simulink model "asbhl20"  (R2016b)
settings: Solver=ode3  StartTime=0.0  StopTime=61  FixedStep=1/120  RelTol=1e-3  AbsTol=1e-6
PreLoadFcn:
  | load asbhl20data.mat
InitFcn:
  | timeSince1970.Value = etime(datevec(now),[1970, 1, 1, 0, 0, 0]);
values from neighbouring files (symbols this model uses):
  maxPackets = 100    [asbhl20data.mat]
  Tc = 0.0166666666667    [asbhl20GlobalChildrenData.mat]
  x_cg = 4.78635044684    [asbhl20data.mat]
undefined symbols (not defined in the file or in its folder): m, message, Receive, s, Send, sigbuilder_block
libraries: aerolibfltsims x5, simulink x4, asbhl20GPS x2, aerolibnav x2, asbhl20env x1, asbhl20airdata x1, asbhl20ralt x1, asbhl20commsys x1, asbhl20FADEC x1, asbhl20sensors x1, asbhl20LGC x1, asbhl20vehicle x1
(part 2 of 3)

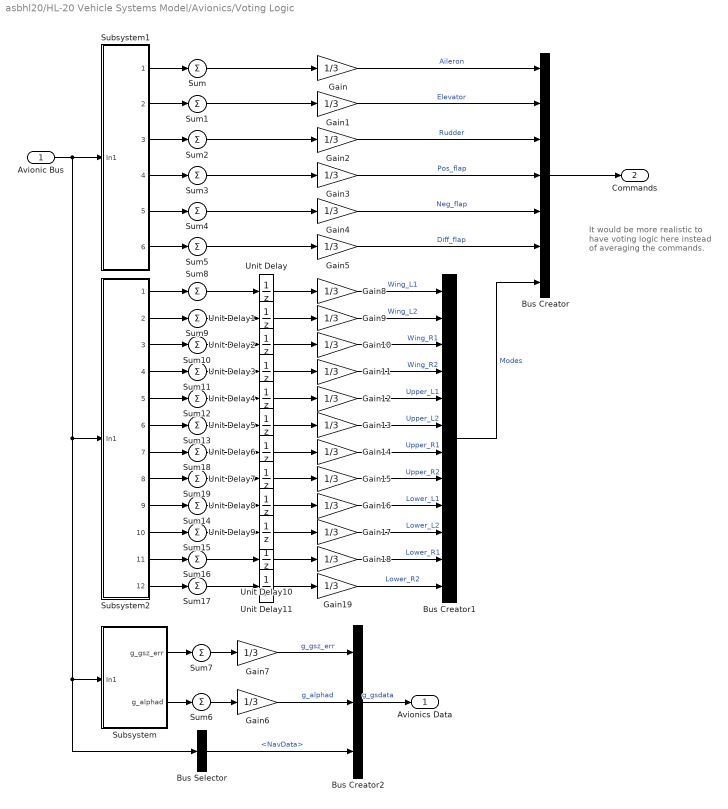
== system asbhl20/HL-20 Vehicle Systems Model/Avionics/Voting Logic ==
  note: It would be more realistic
      | to have voting logic here
      | instead of averaging the
      | commands.
  Avionic Bus : Inport
  Bus Creator : BusCreator  Inputs=7
  Bus Creator1 : BusCreator  Inputs=12
  Bus Creator2 : BusCreator  Inputs=3
  Bus Selector : BusSelector  OutputSignals=Bus1.CPU_A.NavData
  Gain{,1..7} (8 alike) : Gain  Gain=1/3  SaturateOnIntegerOverflow=on  OutDataTypeStr=Inherit: Same as input  ParamDataTypeStr=Inherit: Same as input
  Gain{8..19} (12 alike) : Gain  Gain=1/3  ParamDataTypeStr=float('double')  SaturateOnIntegerOverflow=on  OutDataTypeStr=Inherit: Same as input
  Subsystem : Subsystem
  Subsystem1 : Subsystem
  Subsystem2 : Subsystem
  Sum{,1..19} (20 alike) : Sum  Inputs=+  SaturateOnIntegerOverflow=on
  Unit Delay{,1..11} (12 alike) : UnitDelay  InitialCondition=12  SampleTime=Tc
  Avionics Data : Outport
  Commands : Outport  Port=2
  wires:
  Bus Creator1/1 -> Bus Creator/7  "Modes"
  Gain19/1 -> Bus Creator1/12  "Lower_R2"
  Gain18/1 -> Bus Creator1/11  "Lower_R1"
  Gain17/1 -> Bus Creator1/10  "Lower_L2"
  Gain16/1 -> Bus Creator1/9  "Lower_L1"
  Gain15/1 -> Bus Creator1/8  "Upper_R2"
  Gain14/1 -> Bus Creator1/7  "Upper_R1"
  Gain13/1 -> Bus Creator1/6  "Upper_L2"
  Gain12/1 -> Bus Creator1/5  "Upper_L1"
  Gain11/1 -> Bus Creator1/4  "Wing_R2"
  Gain10/1 -> Bus Creator1/3  "Wing_R1"
  Gain9/1 -> Bus Creator1/2  "Wing_L2"
  Gain8/1 -> Bus Creator1/1  "Wing_L1"
  Subsystem2/12(Lower_R2) -> Sum17/1
  Subsystem2/11(Lower_R1) -> Sum16/1
  Subsystem2/10(Lower_L2) -> Sum15/1
  Subsystem2/9(Lower_L1) -> Sum14/1
  Subsystem2/8(Upper_R2) -> Sum19/1
  Subsystem2/7(Upper_R1) -> Sum18/1
  Sum17/1 -> Unit Delay11/1
  Sum16/1 -> Unit Delay10/1
  Sum15/1 -> Unit Delay9/1
  Sum14/1 -> Unit Delay8/1
  Sum19/1 -> Unit Delay7/1
  Sum18/1 -> Unit Delay6/1
  Subsystem2/6(Upper_L2) -> Sum13/1
  Subsystem2/5(Upper_L1) -> Sum12/1
  Subsystem2/4(Wing_R2) -> Sum11/1
  Subsystem2/3(Wing_R1) -> Sum10/1
  Subsystem2/2(Wing_L2) -> Sum9/1
  Subsystem2/1(Wing_L1) -> Sum8/1
  Sum13/1 -> Unit Delay5/1
  Sum12/1 -> Unit Delay4/1
  Sum11/1 -> Unit Delay3/1
  Sum10/1 -> Unit Delay2/1
  Sum9/1 -> Unit Delay1/1
  Sum8/1 -> Unit Delay/1
  Subsystem/1("g_gsz_err ") -> Sum7/1
  Sum7/1 -> Gain7/1
  Subsystem/2("g_alphad ") -> Sum6/1
  Sum6/1 -> Gain6/1
  Gain6/1 -> Bus Creator2/2  "g_alphad"
  Gain7/1 -> Bus Creator2/1  "g_gsz_err"
  Bus Creator2/1 -> Avionics Data/1  "g_gsdata"
  Subsystem1/4(Pos Flap) -> Sum3/1
  Subsystem1/5(Neg Flap) -> Sum4/1
  Subsystem1/6(Diff Flap) -> Sum5/1
  Bus Creator/1 -> Commands/1
  Gain5/1 -> Bus Creator/6  "Diff_flap"
  Gain4/1 -> Bus Creator/5  "Neg_flap"
  Gain3/1 -> Bus Creator/4  "Pos_flap"
  Sum5/1 -> Gain5/1
  Sum4/1 -> Gain4/1
  Sum3/1 -> Gain3/1
  Gain2/1 -> Bus Creator/3  "Rudder"
  Subsystem1/3(Rudder) -> Sum2/1
  Sum2/1 -> Gain2/1
  Gain1/1 -> Bus Creator/2  "Elevator"
  Subsystem1/2(Elevator) -> Sum1/1
  Sum1/1 -> Gain1/1
  Subsystem1/1(Aileron) -> Sum/1
  Sum/1 -> Gain/1
  Avionic Bus/1 -> Subsystem2/1(In1), Subsystem/1(In1), Bus Selector/1, Subsystem1/1(In1)
  Gain/1 -> Bus Creator/1  "Aileron"
  Bus Selector/1 -> Bus Creator2/3  "<NavData>"
  Unit Delay/1 -> Gain8/1
  Unit Delay1/1 -> Gain9/1
  Unit Delay2/1 -> Gain10/1
  Unit Delay3/1 -> Gain11/1
  Unit Delay4/1 -> Gain12/1
  Unit Delay5/1 -> Gain13/1
  Unit Delay6/1 -> Gain14/1
  Unit Delay7/1 -> Gain15/1
  Unit Delay8/1 -> Gain16/1
  Unit Delay9/1 -> Gain17/1
  Unit Delay10/1 -> Gain18/1
  Unit Delay11/1 -> Gain19/1

== system asbhl20/Viewer and Feedback/FlightGear/Conditionally Receive net_ctrl Packet from FlightGear ==
  note: If FlightGear is not present or becomes unavailable, switch to pre-recorded data to avoid slowing the simulation due to repeated timeouts waiting for data that will not become available.
  Assertion : Assertion  AssertionFailFcn=warning(message('aeroblks:asbhl20:FGMaxPacketsLost'))  StopWhenAssertionFail=off
  Compare To Zero : simulink/Logic and Bit Operations/Compare To Zero  relop===  OutDataTypeStr=boolean
  Ground : Ground
  Memory : Memory  InheritSampleTime=on
  Pre-saved FlightGear data : Subsystem
      mask Display: port_label('output',1,sprintf('FG_data\n(Pre-saved)'))
  Self enabled subsystem receiving FlighGear data : Subsystem  TreatAsAtomicUnit=on
  Switch : Switch  Criteria=u2 ~= 0
  Switch1 : Switch  Criteria=u2 > Threshold
  Trigger a Warning Upon Loss of Connection : Logic  Operator=NAND  IconShape=distinctive  AllPortsSameDT=off  OutDataTypeStr=boolean
  Trigger signal : DiscretePulseGenerator  Period=4  SampleTime=1/120
  Env Data : Outport
  wires:
  Pre-saved FlightGear data/1(FG_data (Pre-saved)) -> Switch/1
  Switch/1 -> Env Data/1
  Compare To Zero/1 -> Trigger a Warning Upon Loss of Connection/1
  Memory/1 -> Compare To Zero/1, Switch1/2
  Ground/1 -> Switch1/1
  Switch1/1 -> Self enabled subsystem receiving FlighGear data/Trigger
  Trigger signal/1 -> Switch1/3
  Self enabled subsystem receiving FlighGear data/2(FGData) -> Switch/3
  Self enabled subsystem receiving FlighGear data/1(LostConn) -> Trigger a Warning Upon Loss of Connection/2, Memory/1, Switch/2
  Trigger a Warning Upon Loss of Connection/1 -> Assertion/1

== system asbhl20/Viewer and Feedback/FlightGear/phidot thetadot psidot ==
  pqr : Inport
  phi theta psi : Inport  Port=2
  Concatenate1 : Concatenate  NumInputs=3
  Concatenate2 : Concatenate  NumInputs=3
  SinCos : aerolibobsolete/SinCos
  phidot : Fcn  Expr=u[1]+(u[2]*u[4]+u[3]*u[7])*(u[5]/u[8])
  psidot : Fcn  Expr=(u[2]*u[4]+u[3]*u[7])/u[8]
  thetadot : Fcn  Expr=u[2]*u[7]-u[3]*u[4]
  ptp_earth : Outport
  ptp_dot : Outport  Port=2
  wires:
  SinCos/2 -> Concatenate1/3
  SinCos/1 -> Concatenate1/2
  Concatenate2/1 -> ptp_dot/1
  phidot/1 -> Concatenate2/1
  thetadot/1 -> Concatenate2/2
  psidot/1 -> Concatenate2/3
  phi theta psi/1 -> ptp_earth/1, SinCos/1
  pqr/1 -> Concatenate1/1
  Concatenate1/1 -> thetadot/1, phidot/1, psidot/1

== system asbhl20/Viewer and Feedback/Signal Builder/Signal Builder ==
  Demux : Demux  Tag=STV Demux  Outputs=8
  FromWs : FromWorkspace  Tag=STV FromWs  VariableName=tuvar  SampleTime=0
      SigBuilderData=|
      | common.afterFinalStr = 'Extrapolate'
      | common.sampleTime = 0
      | dataSet.timeRange = [0 10]
      | dataSet.name = 'Ramp Hold'
      | sbobj.Groups.Name = 'Ramp Hold'
      | sbobj.Groups.Signals(1).Name = 'wind_speed_kt'
      | sbobj.Groups.Signals(1).XData = [0 10]
      | sbobj.Groups.Signals(1).YData = [0 0]
      | sbobj.Groups.Signals(2).Name = 'wind_dir_deg'
      | sbobj.Groups.Signals(2).XData = [0 10]
      | sbobj.Groups.Signals(2).YData = [0 0]
      | sbobj.Groups.Signals(3).Name = 'turbulence_norm'
      | sbobj.Groups.Signals(3).XData = [0 10]
      | sbobj.Groups.Signals(3).YData = [0 0]
      | sbobj.Groups.Signals(4).Name = 'temp_c'
      | sbobj.Groups.Signals(4).XData = [0 10]
      | sbobj.Groups.Signals(4).YData = [-10 -10]
      | sbobj.Groups.Signals(5).Name = 'press_inhg'
      | sbobj.Groups.Signals(5).XData = [0 10]
      | sbobj.Groups.Signals(5).YData = [29.92 29.92]
      | sbobj.Groups.Signals(6).Name = 'hground'
      | sbobj.Groups.Signals(6).XData = [0 10]
      | sbobj.Groups.Signals(6).YData = [1 1]
      | sbobj.Groups.Signals(7).Name = 'magvar'
      | sbobj.Groups.Signals(7).XData = [0 10]
      | sbobj.Groups.Signals(7).YData = [0 0]
      | sbobj.Groups.Signals(8).Name = 'icing'
      | sbobj.Groups.Signals(8).XData = [0 10]
      | sbobj.Groups.Signals(8).YData = [0 0]
  wind_speed_kt : Outport  Tag=STV Outport
  wind_dir_deg : Outport  Tag=STV Outport  Port=2
  turbulence_norm : Outport  Tag=STV Outport  Port=3
  temp_c : Outport  Tag=STV Outport  Port=4
  press_inhg : Outport  Tag=STV Outport  Port=5
  hground : Outport  Tag=STV Outport  Port=6
  magvar : Outport  Tag=STV Outport  Port=7
  icing : Outport  Tag=STV Outport  Port=8
  wires:
  Demux/8 -> icing/1
  Demux/7 -> magvar/1
  Demux/6 -> hground/1
  Demux/5 -> press_inhg/1
  Demux/4 -> temp_c/1
  Demux/3 -> turbulence_norm/1
  Demux/2 -> wind_dir_deg/1
  Demux/1 -> wind_speed_kt/1
  FromWs/1 -> Demux/1

== system asbhl20/HL-20 Vehicle Systems Model/Avionics/Actuator System Failures /Left Lower Inner ==

== system asbhl20/HL-20 Vehicle Systems Model/Avionics/Actuator System Failures /Left Lower Outer ==

== system asbhl20/HL-20 Vehicle Systems Model/Avionics/Actuator System Failures /Left Upper Inner ==

== system asbhl20/HL-20 Vehicle Systems Model/Avionics/Actuator System Failures /Left Upper Outer ==

== system asbhl20/HL-20 Vehicle Systems Model/Avionics/Actuator System Failures /Right Lower Inner ==

== system asbhl20/HL-20 Vehicle Systems Model/Avionics/Actuator System Failures /Right Lower Outer ==

== system asbhl20/HL-20 Vehicle Systems Model/Avionics/Actuator System Failures /Right Upper Inner ==

== system asbhl20/HL-20 Vehicle Systems Model/Avionics/Actuator System Failures /Right Upper Outer ==

== system asbhl20/HL-20 Vehicle Systems Model/Avionics/Actuator System Failures /Wing H1 ==

== system asbhl20/HL-20 Vehicle Systems Model/Avionics/Actuator System Failures /Wing H2 ==

== system asbhl20/HL-20 Vehicle Systems Model/Avionics/Actuator System Failures /Wing H3 ==

== system asbhl20/HL-20 Vehicle Systems Model/Avionics/Actuator System Failures /Wing H4 ==

== system asbhl20/HL-20 Vehicle Systems Model/Avionics/Actuator System Failures /Wing H5 ==

== system asbhl20/HL-20 Vehicle Systems Model/Avionics/Actuator System Failures /Wing H6 ==

== system asbhl20/HL-20 Vehicle Systems Model/Avionics/Actuator System Failures /Wing H7 ==

== system asbhl20/HL-20 Vehicle Systems Model/Avionics/Actuator System Failures /Wing H8 ==

== system asbhl20/HL-20 Vehicle Systems Model/Avionics/Actuator System Failures /Wing H9 ==

== system asbhl20/HL-20 Vehicle Systems Model/Avionics/Actuator System Failures /Wing Left Inner ==

== system asbhl20/HL-20 Vehicle Systems Model/Avionics/Actuator System Failures /Wing Left Outer ==

== system asbhl20/HL-20 Vehicle Systems Model/Avionics/Actuator System Failures /Wing Right Inner ==

== system asbhl20/HL-20 Vehicle Systems Model/Avionics/Actuator System Failures /Wing Right Outer ==

== system asbhl20/HL-20 Vehicle Systems Model/Avionics/Left Avionics Bay/CPU B ==
  note: TODO: add redundant navigation application
  AirData : Inport
  Bus 2 : Inport  Port=2
  Bus 3 : Inport  Port=3
  Failures : Inport  Port=4
  Bus Creator1 : BusCreator  Inputs=4
  Bus Selector : BusSelector  OutputSignals=IMU2
  Bus Selector1 : BusSelector  OutputSignals=GPS2,h_sens
  Event Logging : Subsystem
  FDIR_Application : ModelReference  ModelNameDialog=asbhl20_FDIRApp  SimulationMode=Normal  ModelReferenceVersion=1.160
  FlightControlSystem_Application : ModelReference  ModelNameDialog=asbhl20_FCSApp  SimulationMode=Normal  ModelReferenceVersion=1.52
  GuidanceSystem_Application : ModelReference  ModelNameDialog=asbhl20_GuidanceApp  SimulationMode=Normal  ModelReferenceVersion=1.121
  IMU & GPS Post Process : Subsystem
  CPU_B_out : Outport
  wires:
  IMU & GPS Post Process/2(Guidance i/p) -> GuidanceSystem_Application/1
  IMU & GPS Post Process/1(Control i/p) -> FlightControlSystem_Application/2
  AirData/1 -> FDIR_Application/2, FlightControlSystem_Application/1, IMU & GPS Post Process/1(AirData)
  GuidanceSystem_Application/1 -> Bus Creator1/3, FlightControlSystem_Application/3  "Guidance"
  FlightControlSystem_Application/1 -> Bus Creator1/2  "Demands"
  Bus Creator1/1 -> CPU_B_out/1  "CPU_B"
  Bus Selector/1 -> IMU & GPS Post Process/2(IMU o/p)  "<IMU2>"
  Bus 3/1 -> Bus Selector/1
  Bus 2/1 -> Bus Selector1/1
  Bus Selector1/1 -> IMU & GPS Post Process/3(GPS o/p)  "<GPS2>"
  FDIR_Application/2 -> Bus Creator1/1  "Modes"
  FDIR_Application/1 -> Event Logging/1(Event_log)
  Failures/1 -> FDIR_Application/1
  Bus Selector1/2 -> IMU & GPS Post Process/4(NavData)  "<h_sens>"
  GuidanceSystem_Application/2 -> FlightControlSystem_Application/4
  GuidanceSystem_Application/3 -> Bus Creator1/4  "gsData"

== system asbhl20/HL-20 Vehicle Systems Model/Avionics/Left Avionics Bay/CPU C ==
  note: TODO: add redundant navigation application
  Airdata System o/p : Inport
  Bus 3 : Inport  Port=2
  Bus 1 : Inport  Port=3
  Failures : Inport  Port=4
  Average values : Subsystem
  Bus Creator1 : BusCreator  Inputs=4
  Bus Selector : BusSelector  OutputSignals=IMU2  OutputAsBus=on
  Bus Selector1 : BusSelector  OutputSignals=IMU1,GPS1,CPU_A.NavData
  Event Logging : Subsystem
  FDIR_Application : ModelReference  ModelNameDialog=asbhl20_FDIRApp  SimulationMode=Normal  ModelReferenceVersion=1.160
  FlightControlSystem_Application : ModelReference  ModelNameDialog=asbhl20_FCSApp  SimulationMode=Normal  ModelReferenceVersion=1.52
  GuidanceSystem_Application : ModelReference  ModelNameDialog=asbhl20_GuidanceApp  SimulationMode=Normal  ModelReferenceVersion=1.121
  IMU & GPS Post Process : Subsystem
  CPU_C_out : Outport
  wires:
  IMU & GPS Post Process/1(Control data) -> FlightControlSystem_Application/2
  Airdata System o/p/1 -> FDIR_Application/2, FlightControlSystem_Application/1, IMU & GPS Post Process/1(AirData)
  GuidanceSystem_Application/1 -> Bus Creator1/3, FlightControlSystem_Application/3  "Guidance"
  FlightControlSystem_Application/1 -> Bus Creator1/2  "Demands"
  Bus Creator1/1 -> CPU_C_out/1  "CPU_C"
  IMU & GPS Post Process/2(Guidance data) -> GuidanceSystem_Application/1
  Bus Selector/1 -> Average values/1(IMU2)
  Bus 3/1 -> Bus Selector/1
  Bus 1/1 -> Bus Selector1/1
  Bus Selector1/2 -> IMU & GPS Post Process/3(GPS o/p)  "<GPS1>"
  Bus Selector1/1 -> Average values/2(IMU1)  "<IMU1>"
  Average values/1(IMUave) -> IMU & GPS Post Process/2(IMU o/p)
  FDIR_Application/2 -> Bus Creator1/1  "Modes"
  FDIR_Application/1 -> Event Logging/1(Event_log)
  Failures/1 -> FDIR_Application/1
  Bus Selector1/3 -> IMU & GPS Post Process/4(NavData)  "<NavData>"
  GuidanceSystem_Application/2 -> FlightControlSystem_Application/4
  GuidanceSystem_Application/3 -> Bus Creator1/4  "gsData"

== system asbhl20/HL-20 Vehicle Systems Model/Avionics/Left Avionics Bay/bus comm delay ==
  note: TODO: resolve Demands as a bus
  curr : Inport
  Bus Creator2 : BusCreator  Inputs=3
  Bus Selector3 : BusSelector  OutputSignals=Demands,Guidance,NavData
  Unit Delay1 : UnitDelay  SampleTime=Tc
  Unit Delay7 : UnitDelay  SampleTime=Tc
  Unit Delay8 : UnitDelay  SampleTime=Tc
  prev : Outport
  wires:
  Unit Delay7/1 -> Bus Creator2/2  "Guidance_out"
  Bus Selector3/2 -> Unit Delay7/1  "<Guidance>"
  curr/1 -> Bus Selector3/1
  Bus Selector3/1 -> Unit Delay8/1  "<Demands>"
  Unit Delay8/1 -> Bus Creator2/1  "Demands"
  Bus Creator2/1 -> prev/1
  Bus Selector3/3 -> Unit Delay1/1  "<NavData>"
  Unit Delay1/1 -> Bus Creator2/3  "NavData"

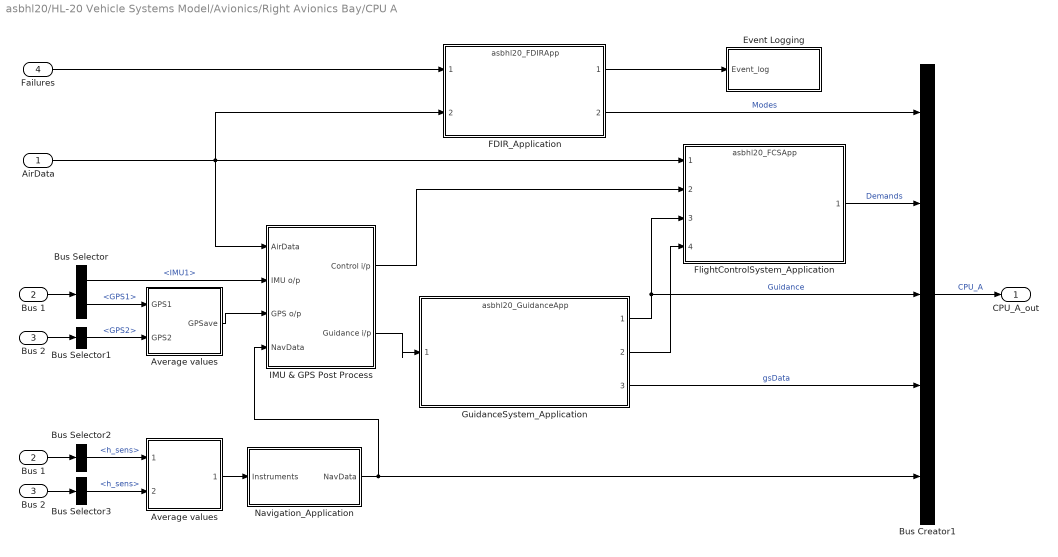
== system asbhl20/HL-20 Vehicle Systems Model/Avionics/Right Avionics Bay/CPU A ==
  AirData : Inport
  Bus 1 : Inport  Port=2
  Bus 2 : Inport  Port=3
  Failures : Inport  Port=4
  Average values : Subsystem
  "Average values " : Subsystem
  Bus Creator1 : BusCreator  Inputs=5
  Bus Selector : BusSelector  OutputSignals=IMU1,GPS1
  Bus Selector1 : BusSelector  OutputSignals=GPS2
  Bus Selector2 : BusSelector  OutputSignals=h_sens
  Bus Selector3 : BusSelector  OutputSignals=h_sens
  "Bus 1 " : InportShadow  Port=2
  "Bus 2 " : InportShadow  Port=3
  Event Logging : Subsystem
  FDIR_Application : ModelReference  ModelNameDialog=asbhl20_FDIRApp  SimulationMode=Normal  ModelReferenceVersion=1.160
  FlightControlSystem_Application : ModelReference  ModelNameDialog=asbhl20_FCSApp  SimulationMode=Normal  ModelReferenceVersion=1.52
  GuidanceSystem_Application : ModelReference  ModelNameDialog=asbhl20_GuidanceApp  SimulationMode=Normal  ModelReferenceVersion=1.121
  IMU & GPS Post Process : Subsystem
  Navigation_Application : Subsystem  TreatAsAtomicUnit=on
  CPU_A_out : Outport
  wires:
  FlightControlSystem_Application/1 -> Bus Creator1/2  "Demands"
  GuidanceSystem_Application/1 -> FlightControlSystem_Application/3, Bus Creator1/3  "Guidance"
  AirData/1 -> IMU & GPS Post Process/1(AirData), FDIR_Application/2, FlightControlSystem_Application/1
  IMU & GPS Post Process/1(Control i/p) -> FlightControlSystem_Application/2
  IMU & GPS Post Process/2(Guidance i/p) -> GuidanceSystem_Application/1
  Bus Creator1/1 -> CPU_A_out/1  "CPU_A"
  Bus Selector/1 -> IMU & GPS Post Process/2(IMU o/p)  "<IMU1>"
  Bus 1/1 -> Bus Selector/1
  Bus 2/1 -> Bus Selector1/1
  Bus Selector1/1 -> Average values/2(GPS2)  "<GPS2>"
  Average values/1(GPSave) -> IMU & GPS Post Process/3(GPS o/p)
  Bus Selector/2 -> Average values/1(GPS1)  "<GPS1>"
  "Bus 1 "/1 -> Bus Selector2/1
  "Bus 2 "/1 -> Bus Selector3/1
  Bus Selector2/1 -> "Average values "/1(h_sens1)  "<h_sens>"
  Bus Selector3/1 -> "Average values "/2(h_sens2)  "<h_sens>"
  "Average values "/1(h_sens_avg) -> Navigation_Application/1(Instruments)
  Navigation_Application/1(NavData) -> Bus Creator1/5, IMU & GPS Post Process/4(NavData)
  FDIR_Application/2 -> Bus Creator1/1  "Modes"
  FDIR_Application/1 -> Event Logging/1(Event_log)
  Failures/1 -> FDIR_Application/1
  GuidanceSystem_Application/2 -> FlightControlSystem_Application/4
  GuidanceSystem_Application/3 -> Bus Creator1/4  "gsData"

== system asbhl20/HL-20 Vehicle Systems Model/Avionics/Right Avionics Bay/bus comm delay ==
  note: TODO: resolve Demands as a bus
  curr : Inport
  Bus Creator2 : BusCreator  Inputs=2
  Bus Selector3 : BusSelector  OutputSignals=Demands,Guidance
  Unit Delay7 : UnitDelay  SampleTime=Tc
  Unit Delay8 : UnitDelay  SampleTime=Tc
  prev : Outport
  wires:
  Unit Delay7/1 -> Bus Creator2/2  "Guidance_out"
  Bus Selector3/2 -> Unit Delay7/1  "<Guidance>"
  curr/1 -> Bus Selector3/1
  Bus Selector3/1 -> Unit Delay8/1  "<Demands>"
  Unit Delay8/1 -> Bus Creator2/1  "Demands"
  Bus Creator2/1 -> prev/1

== system asbhl20/HL-20 Vehicle Systems Model/Avionics/Voting Logic/Subsystem ==
  In1 : Inport
  Bus Selector1 : BusSelector  OutputSignals=Bus1.CPU_A.gsData,Bus2.CPU_B.gsData,Bus3.CPU_C.gsData
  Bus to Vector : BusToVector
  Bus to Vector1 : BusToVector
  Bus to Vector2 : BusToVector
  Mux9 : Mux  Inputs=[2 2 2]
  g_alphad : Selector  InputPortWidth=6  IndexOptions=Index vector (dialog)  Indices=[2 4 6]  OutputSizes=1
  g_gsz_err : Selector  InputPortWidth=6  IndexOptions=Index vector (dialog)  Indices=[1 3 5]  OutputSizes=1
  "g_gsz_err " : Outport
  "g_alphad " : Outport  Port=2
  wires:
  g_alphad/1 -> "g_alphad "/1
  In1/1 -> Bus Selector1/1
  g_gsz_err/1 -> "g_gsz_err "/1
  Bus Selector1/1 -> Bus to Vector/1  "<gsData>"
  Bus Selector1/3 -> Bus to Vector2/1  "<gsData>"
  Bus Selector1/2 -> Bus to Vector1/1  "<gsData>"
  Mux9/1 -> g_alphad/1, g_gsz_err/1
  Bus to Vector/1 -> Mux9/1
  Bus to Vector1/1 -> Mux9/2
  Bus to Vector2/1 -> Mux9/3

== system asbhl20/HL-20 Vehicle Systems Model/Avionics/Voting Logic/Subsystem1 ==
  In1 : Inport
  Bus Selector1 : BusSelector  OutputSignals=Bus1.CPU_A.Demands.Aileron_demand,Bus2.CPU_B.Demands.Aileron_demand,Bus3.CPU_C.Demands.Aileron_demand,Bus1.CPU_A.Demands.Elevator_demand,Bus2.CPU_B.Demands.Elevator_demand,Bus3.CPU_C.Demands.Elevator_demand,Bus1.CPU_A.Demands.Rudder_demand,Bus2.CPU_B.Demands.Rudder_demand,Bus3.CPU_C.Demands.Rudder_demand,Bus1.CPU_A.Demands.Positive_flap_demand,Bus2.CPU_B.Demands.Positive_flap_demand,Bus3.CPU_C.Demands.Positive_flap_demand,Bus1.CPU_A.Demands.Negative_flap_demand,Bus2.CPU_B.Demands.Negative_flap_demand,Bus3.CPU_C.Demands.Negative_flap_demand,Bus1.CPU_A.Demands.Differential_flap_demand,Bus2.CPU_B.Demands.Differential_flap_demand,Bus3.CPU_C.Demands.Differential_flap_demand
  Mux{,1..5} (6 alike) : Mux  Inputs=3
  Aileron : Outport
  Elevator : Outport  Port=2
  Rudder : Outport  Port=3
  Pos Flap : Outport  Port=4
  Neg Flap : Outport  Port=5
  Diff Flap : Outport  Port=6
  wires:
  Mux5/1 -> Diff Flap/1
  Mux4/1 -> Neg Flap/1
  Mux3/1 -> Pos Flap/1
  In1/1 -> Bus Selector1/1
  Mux2/1 -> Rudder/1
  Mux1/1 -> Elevator/1
  Mux/1 -> Aileron/1
  Bus Selector1/1 -> Mux/1  "<Aileron_demand>"
  Bus Selector1/2 -> Mux/2  "<Aileron_demand>"
  Bus Selector1/3 -> Mux/3  "<Aileron_demand>"
  Bus Selector1/4 -> Mux1/1  "<Elevator_demand>"
  Bus Selector1/5 -> Mux1/2  "<Elevator_demand>"
  Bus Selector1/6 -> Mux1/3  "<Elevator_demand>"
  Bus Selector1/7 -> Mux2/1  "<Rudder_demand>"
  Bus Selector1/8 -> Mux2/2  "<Rudder_demand>"
  Bus Selector1/9 -> Mux2/3  "<Rudder_demand>"
  Bus Selector1/10 -> Mux3/1  "<Positive_flap_demand>"
  Bus Selector1/11 -> Mux3/2  "<Positive_flap_demand>"
  Bus Selector1/12 -> Mux3/3  "<Positive_flap_demand>"
  Bus Selector1/13 -> Mux4/1  "<Negative_flap_demand>"
  Bus Selector1/14 -> Mux4/2  "<Negative_flap_demand>"
  Bus Selector1/15 -> Mux4/3  "<Negative_flap_demand>"
  Bus Selector1/16 -> Mux5/1  "<Differential_flap_demand>"
  Bus Selector1/17 -> Mux5/2  "<Differential_flap_demand>"
  Bus Selector1/18 -> Mux5/3  "<Differential_flap_demand>"

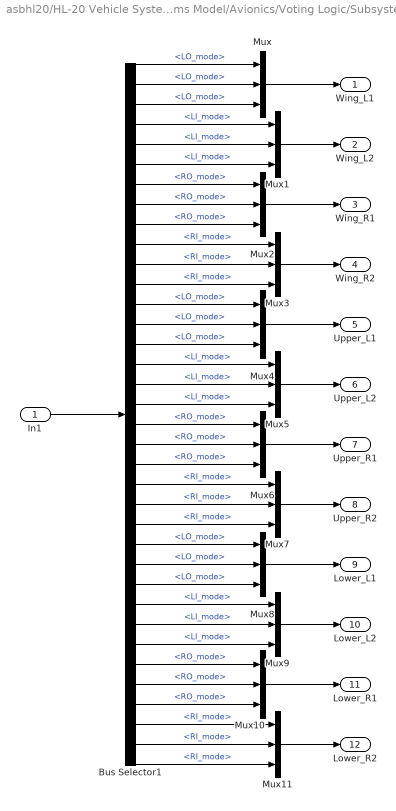
== system asbhl20/HL-20 Vehicle Systems Model/Avionics/Voting Logic/Subsystem2 ==
  In1 : Inport
  Bus Selector1 : BusSelector  OutputSignals=Bus1.CPU_A.Modes.Wing.LO_mode,Bus2.CPU_B.Modes.Wing.LO_mode,Bus3.CPU_C.Modes.Wing.LO_mode,Bus1.CPU_A.Modes.Wing.LI_mode,Bus2.CPU_B.Modes.Wing.LI_mode,Bus3.CPU_C.Modes.Wing.LI_mode,Bus1.CPU_A.Modes.Wing.RO_mode,Bus2.CPU_B.Modes.Wing.RO_mode,Bus3.CPU_C.Modes.Wing.RO_mode,Bus1.CPU_A.Modes.Wing.RI_mode,Bus2.CPU_B.Modes.Wing.RI_mode,Bus3.CPU_C.Modes.Wing.RI_mode,Bus1.CPU_A.Modes.Upper.LO_mode,Bus2.CPU_B.Modes.Upper.LO_mode,Bus3.CPU_C.Modes.Upper.LO_mode,Bus1.CPU_A.Modes.Upper.LI_mode,Bus2.CPU_B.Modes.Upper.LI_mode,Bus3.CPU_C.Modes.Upper.LI_mode,Bus1.CPU_A.Modes.Upper.RO_mode,Bus2.CPU_B.Modes.Upper.RO_mode,Bus3.CPU_C.Modes.Upper.RO_mode,Bus1.CPU_A.Modes.Upper.RI_mode,Bus2.CPU_B.Modes.Upper.RI_mode,Bus3.CPU_C.Modes.Upper.RI_mode,Bus1.CPU_A.Modes.Lower.LO_mode,Bus2.CPU_B.Modes.Lower.LO_mode,Bus3.CPU_C.Modes.Lower.LO_mode,Bus1.CPU_A.Modes.Lower.LI_mode,Bus2.CPU_B.Modes.Lower.LI_mode,Bus3.CPU_C.Modes.Lower.LI_mode,Bus1.CPU_A.Modes.Lower.RO_mode,Bus2.CPU_B.Modes.Lower.RO_mode,Bus3.CPU_C.Modes.Lower.RO_mode,Bus1.CPU_A.Modes.Lower.RI_mode,Bus2.CPU_B.Modes.Lower.RI_mode,Bus3.CPU_C.Modes.Lower.RI_mode
  Mux{,1..11} (12 alike) : Mux  Inputs=3
  Wing_L1 : Outport
  Wing_L2 : Outport  Port=2
  Wing_R1 : Outport  Port=3
  Wing_R2 : Outport  Port=4
  Upper_L1 : Outport  Port=5
  Upper_L2 : Outport  Port=6
  Upper_R1 : Outport  Port=7
  Upper_R2 : Outport  Port=8
  Lower_L1 : Outport  Port=9
  Lower_L2 : Outport  Port=10
  Lower_R1 : Outport  Port=11
  Lower_R2 : Outport  Port=12
  wires:
  Mux11/1 -> Lower_R2/1
  Mux10/1 -> Lower_R1/1
  Mux9/1 -> Lower_L2/1
  Mux8/1 -> Lower_L1/1
  Mux7/1 -> Upper_R2/1
  Mux6/1 -> Upper_R1/1
  Bus Selector1/36 -> Mux11/3  "<RI_mode>"
  Bus Selector1/35 -> Mux11/2  "<RI_mode>"
  Bus Selector1/34 -> Mux11/1  "<RI_mode>"
  Bus Selector1/33 -> Mux10/3  "<RO_mode>"
  Bus Selector1/32 -> Mux10/2  "<RO_mode>"
  Bus Selector1/31 -> Mux10/1  "<RO_mode>"
  Bus Selector1/30 -> Mux9/3  "<LI_mode>"
  Bus Selector1/29 -> Mux9/2  "<LI_mode>"
  Bus Selector1/28 -> Mux9/1  "<LI_mode>"
  Bus Selector1/27 -> Mux8/3  "<LO_mode>"
  Bus Selector1/26 -> Mux8/2  "<LO_mode>"
  Bus Selector1/25 -> Mux8/1  "<LO_mode>"
  Bus Selector1/24 -> Mux7/3  "<RI_mode>"
  Bus Selector1/23 -> Mux7/2  "<RI_mode>"
  Bus Selector1/22 -> Mux7/1  "<RI_mode>"
  Bus Selector1/21 -> Mux6/3  "<RO_mode>"
  Bus Selector1/20 -> Mux6/2  "<RO_mode>"
  Bus Selector1/19 -> Mux6/1  "<RO_mode>"
  Bus Selector1/18 -> Mux5/3  "<LI_mode>"
  Bus Selector1/17 -> Mux5/2  "<LI_mode>"
  Bus Selector1/16 -> Mux5/1  "<LI_mode>"
  Bus Selector1/15 -> Mux4/3  "<LO_mode>"
  Bus Selector1/14 -> Mux4/2  "<LO_mode>"
  Bus Selector1/13 -> Mux4/1  "<LO_mode>"
  Bus Selector1/12 -> Mux3/3  "<RI_mode>"
  Bus Selector1/11 -> Mux3/2  "<RI_mode>"
  Bus Selector1/10 -> Mux3/1  "<RI_mode>"
  Bus Selector1/9 -> Mux2/3  "<RO_mode>"
  Bus Selector1/8 -> Mux2/2  "<RO_mode>"
  Bus Selector1/7 -> Mux2/1  "<RO_mode>"
  Bus Selector1/6 -> Mux1/3  "<LI_mode>"
  Bus Selector1/5 -> Mux1/2  "<LI_mode>"
  Bus Selector1/4 -> Mux1/1  "<LI_mode>"
  Bus Selector1/3 -> Mux/3  "<LO_mode>"
  Bus Selector1/2 -> Mux/2  "<LO_mode>"
  Bus Selector1/1 -> Mux/1  "<LO_mode>"
  Mux/1 -> Wing_L1/1
  Mux1/1 -> Wing_L2/1
  Mux2/1 -> Wing_R1/1
  In1/1 -> Bus Selector1/1
  Mux3/1 -> Wing_R2/1
  Mux4/1 -> Upper_L1/1
  Mux5/1 -> Upper_L2/1

== system asbhl20/Viewer and Feedback/FlightGear/Conditionally Receive net_ctrl Packet from FlightGear/Pre-saved FlightGear data ==
  Bus Creator2 : BusCreator  Inputs=8  OutDataTypeStr=Bus: FlightGearBus
  Data Type Conversion : DataTypeConversion  OutDataTypeStr=uint32
  Demux2 : Demux  Outputs=8
  From File : FromFile  FileName=asbhl20FlightGear.mat  SampleTime=1/120
  FG_data (Pre-saved) : Outport
  wires:
  From File/1 -> Demux2/1
  Demux2/6 -> Bus Creator2/6  "hground"
  Data Type Conversion/1 -> Bus Creator2/8  "icing"
  Demux2/7 -> Bus Creator2/7  "magvar"
  Demux2/4 -> Bus Creator2/4  "temp_c"
  Demux2/3 -> Bus Creator2/3  "turbulence_norm"
  Demux2/2 -> Bus Creator2/2  "wind_dir_deg"
  Demux2/1 -> Bus Creator2/1  "wind_speed_kt"
  Demux2/8 -> Data Type Conversion/1
  Demux2/5 -> Bus Creator2/5  "press_inhg"
  Bus Creator2/1 -> FG_data (Pre-saved)/1

== system asbhl20/Viewer and Feedback/FlightGear/Conditionally Receive net_ctrl Packet from FlightGear/Self enabled subsystem receiving FlighGear data ==
  Trigger : TriggerPort  VariantControl=Variant
  Bias : Bias  Bias=1
  Bus Creator1 : BusCreator  Inputs=8  OutDataTypeStr=Bus: FlightGearBus
  Compare To Constant : simulink/Logic and Bit Operations/Compare To Constant  relop=>=  const=maxPackets  OutDataTypeStr=boolean
  Constant : Constant  Value=0
  Memory : Memory  InheritSampleTime=on
  Receive net_ctrl Packet from FlightGear : aerolibfltsims/Receive net_ctrl Packet from FlightGear  FlightGearVersion=v2016.1  ReceiveAddress=127.0.0.1  ReceivePort=5505  ReceiveWidth=744  varLen=off  SampleTime=-1  packetFlag=on
      settings: AttributesFormatString=Version Selected:\n%<FlightGearVersion>
  Switch : Switch  Criteria=u2 > Threshold
  Unpack net_ctrl Packet from FlightGear : aerolibfltsims/Unpack net_ctrl Packet from FlightGear  FlightGearVersion=v2016.1  ShowControlSurfacePositionOutputs=off  ShowEngineFuelOutputs=off  ShowLandingGearOutputs=off  ShowAvionicOutputs=off  ShowEnvironmentOutputs=on  SampleTime=-1
      settings: AttributesFormatString=Version Selected: %<FlightGearVersion>
  LostConn : Outport  InitialOutput=0
  FGData : Outport  Port=2
  wires:
  Receive net_ctrl Packet from FlightGear/2 -> Switch/2
  Switch/1 -> Memory/1, Compare To Constant/1
  Bias/1 -> Switch/3
  Constant/1 -> Switch/1
  Memory/1 -> Bias/1
  Compare To Constant/1 -> LostConn/1
  Unpack net_ctrl Packet from FlightGear/6 -> Bus Creator1/6  "hground"
  Unpack net_ctrl Packet from FlightGear/8 -> Bus Creator1/8  "icing"
  Unpack net_ctrl Packet from FlightGear/7 -> Bus Creator1/7  "magvar"
  Unpack net_ctrl Packet from FlightGear/5 -> Bus Creator1/5  "press_inhg"
  Unpack net_ctrl Packet from FlightGear/4 -> Bus Creator1/4  "temp_c"
  Unpack net_ctrl Packet from FlightGear/3 -> Bus Creator1/3  "turbulence_norm"
  Unpack net_ctrl Packet from FlightGear/2 -> Bus Creator1/2  "wind_dir_deg"
  Unpack net_ctrl Packet from FlightGear/1 -> Bus Creator1/1  "wind_speed_kt"
  Receive net_ctrl Packet from FlightGear/1 -> Unpack net_ctrl Packet from FlightGear/1
  Bus Creator1/1 -> FGData/1

== system asbhl20/HL-20 Vehicle Systems Model/Avionics/Left Avionics Bay/CPU B/Event Logging ==
  Event_log : Inport
  Bus Selector : BusSelector  OutputSignals=Left_log,Right_log,Wing_log,WingH_log,UpperH_log,LowerH_log
  Event Logging Left : Subsystem
  Event Logging Lower Hydraulic : Subsystem
  Event Logging Right : Subsystem
  Event Logging Upper Hydraulic : Subsystem
  Event Logging Wing : Subsystem
  Event Logging Wing Hydraulic : Subsystem
  wires:
  Event_log/1 -> Bus Selector/1
  Bus Selector/1 -> Event Logging Left/1(In1)  "<Left_log>"
  Bus Selector/2 -> Event Logging Right/1(In1)  "<Right_log>"
  Bus Selector/3 -> Event Logging Wing/1(In1)  "<Wing_log>"
  Bus Selector/4 -> Event Logging Wing Hydraulic/1(In1)  "<WingH_log>"
  Bus Selector/5 -> Event Logging Upper Hydraulic/1(In1)  "<UpperH_log>"
  Bus Selector/6 -> Event Logging Lower Hydraulic/1(In1)  "<LowerH_log>"

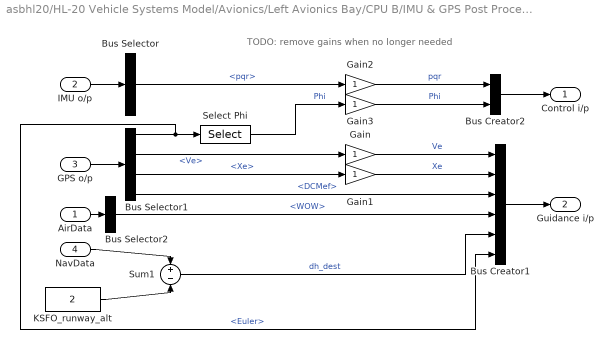
== system asbhl20/HL-20 Vehicle Systems Model/Avionics/Left Avionics Bay/CPU B/IMU & GPS Post Process ==
  note: TODO: remove gains when no longer needed
  AirData : Inport
  IMU o/p : Inport  Port=2
  GPS o/p : Inport  Port=3
  NavData : Inport  Port=4
  Bus Creator1 : BusCreator  Inputs=6  OutDataTypeStr=Bus: GuidanceBus
  Bus Creator2 : BusCreator  Inputs=2  OutDataTypeStr=Bus: FCSSensorBus
  Bus Selector : BusSelector  OutputSignals=pqr
  Bus Selector1 : BusSelector  OutputSignals=Euler,Ve,Xe,DCMef
  Bus Selector2 : BusSelector  OutputSignals=WOW
  Gain{,1..3} (4 alike) : Gain
  KSFO_runway_alt : Constant  Value=2  SampleTime=Tc
  Select Phi : Selector  InputPortWidth=3  IndexOptions=Index vector (dialog)  Indices=[1]  OutputSizes=1
  Sum1 : Sum  Inputs=+-
  Control i/p : Outport
  Guidance i/p : Outport  Port=2
  wires:
  GPS o/p/1 -> Bus Selector1/1
  IMU o/p/1 -> Bus Selector/1
  Bus Creator1/1 -> Guidance i/p/1
  Select Phi/1 -> Gain3/1  "Phi"
  Bus Creator2/1 -> Control i/p/1
  Bus Selector/1 -> Gain2/1  "<pqr>"
  Bus Selector1/3 -> Gain1/1  "<Xe>"
  Bus Selector1/1 -> Select Phi/1, Bus Creator1/6  "<Euler>"
  Bus Selector1/2 -> Gain/1  "<Ve>"
  AirData/1 -> Bus Selector2/1
  Bus Selector2/1 -> Bus Creator1/4  "<WOW>"
  Gain/1 -> Bus Creator1/1  "Ve"
  Gain1/1 -> Bus Creator1/2  "Xe"
  Gain2/1 -> Bus Creator2/1  "pqr"
  Gain3/1 -> Bus Creator2/2  "Phi"
  Bus Selector1/4 -> Bus Creator1/3  "<DCMef>"
  NavData/1 -> Sum1/1
  Sum1/1 -> Bus Creator1/5  "dh_dest"
  KSFO_runway_alt/1 -> Sum1/2

== system asbhl20/HL-20 Vehicle Systems Model/Avionics/Left Avionics Bay/CPU C/Average values ==
  IMU2 : Inport
  IMU1 : Inport  Port=2
  Bus Creator1 : BusCreator  Inputs=1
  Bus Selector : BusSelector  OutputSignals=pqr
  Bus Selector1 : BusSelector  OutputSignals=pqr
  Gain : Gain  Gain=0.5  SaturateOnIntegerOverflow=on  OutDataTypeStr=Inherit: Same as input  ParamDataTypeStr=Inherit: Same as input
  Sum : Sum  Inputs=+|+  SaturateOnIntegerOverflow=on
  IMUave : Outport
  wires:
  IMU1/1 -> Bus Selector/1
  Sum/1 -> Gain/1
  IMU2/1 -> Bus Selector1/1
  Bus Selector1/1 -> Sum/1  "<pqr>"
  Bus Selector/1 -> Sum/2  "<pqr>"
  Gain/1 -> Bus Creator1/1  "pqr"
  Bus Creator1/1 -> IMUave/1

== system asbhl20/HL-20 Vehicle Systems Model/Avionics/Left Avionics Bay/CPU C/Event Logging ==
  Event_log : Inport
  Bus Selector : BusSelector  OutputSignals=Left_log,Right_log,Wing_log,WingH_log,UpperH_log,LowerH_log
  Event Logging Left : Subsystem
  Event Logging Lower Hydraulic : Subsystem
  Event Logging Right : Subsystem
  Event Logging Upper Hydraulic : Subsystem
  Event Logging Wing : Subsystem
  Event Logging Wing Hydraulic : Subsystem
  wires:
  Event_log/1 -> Bus Selector/1
  Bus Selector/1 -> Event Logging Left/1(In1)  "<Left_log>"
  Bus Selector/2 -> Event Logging Right/1(In1)  "<Right_log>"
  Bus Selector/3 -> Event Logging Wing/1(In1)  "<Wing_log>"
  Bus Selector/4 -> Event Logging Wing Hydraulic/1(In1)  "<WingH_log>"
  Bus Selector/5 -> Event Logging Upper Hydraulic/1(In1)  "<UpperH_log>"
  Bus Selector/6 -> Event Logging Lower Hydraulic/1(In1)  "<LowerH_log>"

== system asbhl20/HL-20 Vehicle Systems Model/Avionics/Left Avionics Bay/CPU C/IMU & GPS Post Process ==
  note: TODO: resolve signals without gain-of-1
  AirData : Inport
  IMU o/p : Inport  Port=2
  GPS o/p : Inport  Port=3
  NavData : Inport  Port=4
  Bus Creator2 : BusCreator  Inputs=2  OutDataTypeStr=Bus: FCSSensorBus
  Bus Creator3 : BusCreator  Inputs=6  OutDataTypeStr=Bus: GuidanceBus
  Bus Selector : BusSelector  OutputSignals=pqr
  Bus Selector1 : BusSelector  OutputSignals=Euler,Ve,Xe,DCMef
  Bus Selector2 : BusSelector  OutputSignals=WOW
  Bus Selector3 : BusSelector  OutputSignals=dh_dest
  Gain{,1..3} (4 alike) : Gain
  Select Phi : Selector  InputPortWidth=3  IndexOptions=Index vector (dialog)  Indices=[1]  OutputSizes=1
  Control data : Outport
  Guidance data : Outport  Port=2
  wires:
  GPS o/p/1 -> Bus Selector1/1
  IMU o/p/1 -> Bus Selector/1
  Bus Creator3/1 -> Guidance data/1
  Select Phi/1 -> Gain3/1  "Phi"
  Bus Creator2/1 -> Control data/1
  Bus Selector/1 -> Gain2/1  "<pqr>"
  Bus Selector1/3 -> Gain1/1  "<Xe>"
  Bus Selector1/1 -> Bus Creator3/6, Select Phi/1  "<Euler>"
  Bus Selector1/2 -> Gain/1  "<Ve>"
  AirData/1 -> Bus Selector2/1
  Bus Selector2/1 -> Bus Creator3/4  "<WOW>"
  Gain/1 -> Bus Creator3/1  "Ve"
  Gain1/1 -> Bus Creator3/2  "Xe"
  Gain2/1 -> Bus Creator2/1  "pqr"
  Gain3/1 -> Bus Creator2/2  "Phi"
  Bus Selector1/4 -> Bus Creator3/3  "<DCMef>"
  NavData/1 -> Bus Selector3/1
  Bus Selector3/1 -> Bus Creator3/5  "<dh_dest>"

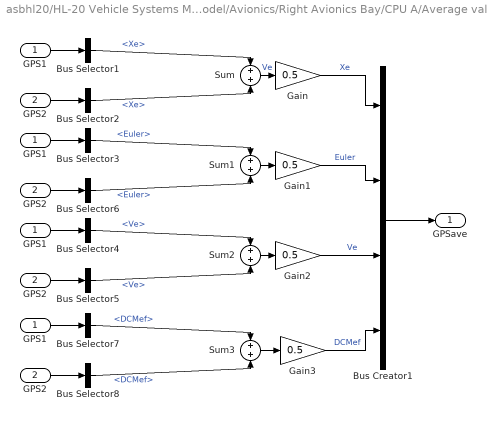
== system asbhl20/HL-20 Vehicle Systems Model/Avionics/Right Avionics Bay/CPU A/Average values ==
  GPS1 : Inport
  GPS2 : Inport  Port=2
  " GPS1" : InportShadow
  " GPS1 " : InportShadow
  " GPS2" : InportShadow  Port=2
  " GPS2 " : InportShadow  Port=2
  Bus Creator1 : BusCreator  Inputs=4
  Bus Selector1 : BusSelector  OutputSignals=Xe
  Bus Selector2 : BusSelector  OutputSignals=Xe
  Bus Selector3 : BusSelector  OutputSignals=Euler
  Bus Selector4 : BusSelector  OutputSignals=Ve
  Bus Selector5 : BusSelector  OutputSignals=Ve
  Bus Selector6 : BusSelector  OutputSignals=Euler
  Bus Selector7 : BusSelector  OutputSignals=DCMef
  Bus Selector8 : BusSelector  OutputSignals=DCMef
  "GPS1 " : InportShadow
  "GPS2 " : InportShadow  Port=2
  Gain{,1..3} (4 alike) : Gain  Gain=0.5  SaturateOnIntegerOverflow=on  OutDataTypeStr=Inherit: Same as input  ParamDataTypeStr=Inherit: Same as input
  Sum{,1..3} (4 alike) : Sum  Inputs=+|+  SaturateOnIntegerOverflow=on
  GPSave : Outport
  wires:
  GPS2/1 -> Bus Selector2/1
  Sum/1 -> Gain/1  "Ve"
  GPS1/1 -> Bus Selector1/1
  Bus Creator1/1 -> GPSave/1
  Sum1/1 -> Gain1/1
  Gain1/1 -> Bus Creator1/2  "Euler"
  Gain/1 -> Bus Creator1/1  "Xe"
  Bus Selector1/1 -> Sum/1  "<Xe>"
  Bus Selector2/1 -> Sum/2  "<Xe>"
  Sum2/1 -> Gain2/1
  Gain2/1 -> Bus Creator1/3  "Ve"
  "GPS1 "/1 -> Bus Selector3/1
  Bus Selector3/1 -> Sum1/1  "<Euler>"
  " GPS1"/1 -> Bus Selector4/1
  Bus Selector4/1 -> Sum2/1  "<Ve>"
  " GPS2"/1 -> Bus Selector5/1
  Bus Selector5/1 -> Sum2/2  "<Ve>"
  "GPS2 "/1 -> Bus Selector6/1
  Bus Selector6/1 -> Sum1/2  "<Euler>"
  " GPS1 "/1 -> Bus Selector7/1
  Bus Selector7/1 -> Sum3/1  "<DCMef>"
  " GPS2 "/1 -> Bus Selector8/1
  Bus Selector8/1 -> Sum3/2  "<DCMef>"
  Sum3/1 -> Gain3/1
  Gain3/1 -> Bus Creator1/4  "DCMef"

== system asbhl20/HL-20 Vehicle Systems Model/Avionics/Right Avionics Bay/CPU A/Average values  ==
  h_sens1 : Inport
  h_sens2 : Inport  Port=2
  Gain : Gain  Gain=0.5  SaturateOnIntegerOverflow=on  OutDataTypeStr=Inherit: Same as input  ParamDataTypeStr=Inherit: Same as input
  Sum : Sum  Inputs=+|+  SaturateOnIntegerOverflow=on
  h_sens_avg : Outport
  wires:
  Gain/1 -> h_sens_avg/1  "h_sens_ave"
  h_sens1/1 -> Sum/1
  Sum/1 -> Gain/1
  h_sens2/1 -> Sum/2

== system asbhl20/HL-20 Vehicle Systems Model/Avionics/Right Avionics Bay/CPU A/Event Logging ==
  Event_log : Inport
  Bus Selector : BusSelector  OutputSignals=Left_log,Right_log,Wing_log,WingH_log,UpperH_log,LowerH_log
  Event Logging Left : Subsystem
  Event Logging Lower Hydraulic : Subsystem
  Event Logging Right : Subsystem
  Event Logging Upper Hydraulic : Subsystem
  Event Logging Wing : Subsystem
  Event Logging Wing Hydraulic : Subsystem
  wires:
  Event_log/1 -> Bus Selector/1
  Bus Selector/1 -> Event Logging Left/1(In1)  "<Left_log>"
  Bus Selector/2 -> Event Logging Right/1(In1)  "<Right_log>"
  Bus Selector/3 -> Event Logging Wing/1(In1)  "<Wing_log>"
  Bus Selector/4 -> Event Logging Wing Hydraulic/1(In1)  "<WingH_log>"
  Bus Selector/5 -> Event Logging Upper Hydraulic/1(In1)  "<UpperH_log>"
  Bus Selector/6 -> Event Logging Lower Hydraulic/1(In1)  "<LowerH_log>"

== system asbhl20/HL-20 Vehicle Systems Model/Avionics/Right Avionics Bay/CPU A/IMU & GPS Post Process ==
  note: TODO: resolve signals without gain-of-1
  AirData : Inport
  IMU o/p : Inport  Port=2
  GPS o/p : Inport  Port=3
  NavData : Inport  Port=4
  Bus Creator1 : BusCreator  Inputs=6  OutDataTypeStr=Bus: GuidanceBus
  Bus Creator2 : BusCreator  Inputs=2  OutDataTypeStr=Bus: FCSSensorBus
  Bus Selector : BusSelector  OutputSignals=pqr
  Bus Selector1 : BusSelector  OutputSignals=Euler,Ve,Xe,DCMef
  Bus Selector2 : BusSelector  OutputSignals=WOW
  Bus Selector3 : BusSelector  OutputSignals=dh_dest
  Gain : Gain
  Gain1 : Gain
  Select Phi : Selector  InputPortWidth=3  IndexOptions=Index vector (dialog)  Indices=[1]  OutputSizes=1
  Control i/p : Outport
  Guidance i/p : Outport  Port=2
  wires:
  GPS o/p/1 -> Bus Selector1/1
  IMU o/p/1 -> Bus Selector/1
  Bus Creator1/1 -> Guidance i/p/1
  Select Phi/1 -> Gain1/1
  Bus Creator2/1 -> Control i/p/1
  Bus Selector/1 -> Gain/1  "<pqr>"
  Bus Selector1/3 -> Bus Creator1/2  "<Xe>"
  Bus Selector1/1 -> Bus Creator1/6, Select Phi/1  "<Euler>"
  Bus Selector1/2 -> Bus Creator1/1  "<Ve>"
  AirData/1 -> Bus Selector2/1
  Bus Selector2/1 -> Bus Creator1/4  "<WOW>"
  Gain/1 -> Bus Creator2/1  "pqr"
  Gain1/1 -> Bus Creator2/2  "Phi"
  Bus Selector1/4 -> Bus Creator1/3  "<DCMef>"
  NavData/1 -> Bus Selector3/1
  Bus Selector3/1 -> Bus Creator1/5  "<dh_dest>"

== system asbhl20/HL-20 Vehicle Systems Model/Avionics/Right Avionics Bay/CPU A/Navigation_Application ==
  Instruments : Inport
  Bus Creator2 : BusCreator  Inputs=2
  Gain : Gain
  KSFO_runway_alt : Constant  Value=2  SampleTime=Tc
  Sum : Sum  Inputs=-+
  NavData : Outport
  wires:
  KSFO_runway_alt/1 -> Bus Creator2/1, Sum/1  "h_dest"
  Bus Creator2/1 -> NavData/1  "NavData"
  Sum/1 -> Bus Creator2/2  "dh_dest"
  Instruments/1 -> Gain/1
  Gain/1 -> Sum/2

== system asbhl20/HL-20 Vehicle Systems Model/Avionics/Left Avionics Bay/CPU B/Event Logging/Event Logging Left ==
  In1 : Inport
  Bus Selector : BusSelector  OutputSignals=signal1,signal2,signal3,signal4,signal5.LU1_log,signal5.LU2_log,signal5.LL1_log,signal5.LL2_log
  Log LL1 Actuator Position Sensors : Subsystem  TreatAsAtomicUnit=on
  Log LL2 Actuator Position Sensors : Subsystem  TreatAsAtomicUnit=on
  Log LU1 Actuator Position Sensors : Subsystem  TreatAsAtomicUnit=on
  Log LU2 Actuator Position Sensors : Subsystem  TreatAsAtomicUnit=on
  wires:
  [LU1_log] -> Log LU1 Actuator Position Sensors/Enable
  In1/1 -> Bus Selector/1
  [LU2_log] -> Log LU2 Actuator Position Sensors/Enable
  [LL1_log] -> Log LL1 Actuator Position Sensors/Enable
  [LL2_log] -> Log LL2 Actuator Position Sensors/Enable
  Bus Selector/1 -> Log LU1 Actuator Position Sensors/1(In1)  "<signal1>"
  Bus Selector/2 -> Log LU2 Actuator Position Sensors/1(In1)  "<signal2>"
  Bus Selector/3 -> Log LL1 Actuator Position Sensors/1(In1)  "<signal3>"
  Bus Selector/4 -> Log LL2 Actuator Position Sensors/1(In1)  "<signal4>"
  Bus Selector/5 -> [LU1_log]  "<LU1_log>"
  Bus Selector/6 -> [LU2_log]  "<LU2_log>"
  Bus Selector/7 -> [LL1_log]  "<LL1_log>"
  Bus Selector/8 -> [LL2_log]  "<LL2_log>"

== system asbhl20/HL-20 Vehicle Systems Model/Avionics/Left Avionics Bay/CPU B/Event Logging/Event Logging Lower Hydraulic ==
  In1 : Inport
  Bus Selector : BusSelector  OutputSignals=signal1,signal2,signal3,signal4.H7_log,signal4.H8_log,signal4.H9_log
  Log Hydraulic System 1 Sensors : Subsystem  TreatAsAtomicUnit=on
  Log Hydraulic System 2 Sensors : Subsystem  TreatAsAtomicUnit=on
  Log Hydraulic System 3 Sensors : Subsystem  TreatAsAtomicUnit=on
  wires:
  [H7_log] -> Log Hydraulic System 1 Sensors/Enable
  In1/1 -> Bus Selector/1
  [H8_log] -> Log Hydraulic System 2 Sensors/Enable
  [H9_log] -> Log Hydraulic System 3 Sensors/Enable
  Bus Selector/1 -> Log Hydraulic System 1 Sensors/1(In1)  "<signal1>"
  Bus Selector/2 -> Log Hydraulic System 2 Sensors/1(In1)  "<signal2>"
  Bus Selector/3 -> Log Hydraulic System 3 Sensors/1(In1)  "<signal3>"
  Bus Selector/4 -> [H7_log]  "<H7_log>"
  Bus Selector/5 -> [H8_log]  "<H8_log>"
  Bus Selector/6 -> [H9_log]  "<H9_log>"

== system asbhl20/HL-20 Vehicle Systems Model/Avionics/Left Avionics Bay/CPU B/Event Logging/Event Logging Right ==
  In1 : Inport
  Bus Selector : BusSelector  OutputSignals=signal1,signal2,signal3,signal4,signal5.RU1_log,signal5.RU2_log,signal5.RL1_log,signal5.RL2_log
  Log RL1 Actuator Position Sensors : Subsystem  TreatAsAtomicUnit=on
  Log RL2 Actuator Position Sensors : Subsystem  TreatAsAtomicUnit=on
  Log RU1 Actuator Position Sensors : Subsystem  TreatAsAtomicUnit=on
  Log RU2 Actuator Position Sensors : Subsystem  TreatAsAtomicUnit=on
  wires:
  Bus Selector/4 -> Log RL2 Actuator Position Sensors/1(In1)  "<signal4>"
  Bus Selector/3 -> Log RL1 Actuator Position Sensors/1(In1)  "<signal3>"
  Bus Selector/2 -> Log RU2 Actuator Position Sensors/1(In1)  "<signal2>"
  Bus Selector/1 -> Log RU1 Actuator Position Sensors/1(In1)  "<signal1>"
  [RL2_log] -> Log RL2 Actuator Position Sensors/Enable
  [RL1_log] -> Log RL1 Actuator Position Sensors/Enable
  [RU2_log] -> Log RU2 Actuator Position Sensors/Enable
  In1/1 -> Bus Selector/1
  [RU1_log] -> Log RU1 Actuator Position Sensors/Enable
  Bus Selector/5 -> [RU1_log]  "<RU1_log>"
  Bus Selector/6 -> [RU2_log]  "<RU2_log>"
  Bus Selector/7 -> [RL1_log]  "<RL1_log>"
  Bus Selector/8 -> [RL2_log]  "<RL2_log>"

== system asbhl20/HL-20 Vehicle Systems Model/Avionics/Left Avionics Bay/CPU B/Event Logging/Event Logging Upper Hydraulic ==
  In1 : Inport
  Bus Selector : BusSelector  OutputSignals=signal1,signal2,signal3,signal4.H4_log,signal4.H5_log,signal4.H6_log
  Log Hydraulic System 1 Sensors : Subsystem  TreatAsAtomicUnit=on
  Log Hydraulic System 2 Sensors : Subsystem  TreatAsAtomicUnit=on
  Log Hydraulic System 3 Sensors : Subsystem  TreatAsAtomicUnit=on
  wires:
  Bus Selector/3 -> Log Hydraulic System 3 Sensors/1(In1)  "<signal3>"
  Bus Selector/2 -> Log Hydraulic System 2 Sensors/1(In1)  "<signal2>"
  Bus Selector/1 -> Log Hydraulic System 1 Sensors/1(In1)  "<signal1>"
  [H6_log] -> Log Hydraulic System 3 Sensors/Enable
  [H5_log] -> Log Hydraulic System 2 Sensors/Enable
  In1/1 -> Bus Selector/1
  [H4_log] -> Log Hydraulic System 1 Sensors/Enable
  Bus Selector/4 -> [H4_log]  "<H4_log>"
  Bus Selector/5 -> [H5_log]  "<H5_log>"
  Bus Selector/6 -> [H6_log]  "<H6_log>"

== system asbhl20/HL-20 Vehicle Systems Model/Avionics/Left Avionics Bay/CPU B/Event Logging/Event Logging Wing ==
  In1 : Inport
  Bus Selector1 : BusSelector  OutputSignals=signal1,signal2,signal3,signal4,signal5.WR1_log,signal5.WR2_log,signal5.WL1_log,signal5.WL2_log
  Log WL1 Actuator Position Sensors : Subsystem  TreatAsAtomicUnit=on
  Log WL2 Actuator Position Sensors : Subsystem  TreatAsAtomicUnit=on
  Log WR1 Actuator Position Sensors : Subsystem  TreatAsAtomicUnit=on
  Log WR2 Actuator Position Sensors : Subsystem  TreatAsAtomicUnit=on
  wires:
  [WR1_log] -> Log WR1 Actuator Position Sensors/Enable
  In1/1 -> Bus Selector1/1
  [WR2_log] -> Log WR2 Actuator Position Sensors/Enable
  [WL1_log] -> Log WL1 Actuator Position Sensors/Enable
  [WL2_log] -> Log WL2 Actuator Position Sensors/Enable
  Bus Selector1/1 -> Log WR1 Actuator Position Sensors/1(In1)  "<signal1>"
  Bus Selector1/2 -> Log WR2 Actuator Position Sensors/1(In1)  "<signal2>"
  Bus Selector1/3 -> Log WL1 Actuator Position Sensors/1(In1)  "<signal3>"
  Bus Selector1/4 -> Log WL2 Actuator Position Sensors/1(In1)  "<signal4>"
  Bus Selector1/5 -> [WR1_log]  "<WR1_log>"
  Bus Selector1/6 -> [WR2_log]  "<WR2_log>"
  Bus Selector1/7 -> [WL1_log]  "<WL1_log>"
  Bus Selector1/8 -> [WL2_log]  "<WL2_log>"

== system asbhl20/HL-20 Vehicle Systems Model/Avionics/Left Avionics Bay/CPU B/Event Logging/Event Logging Wing Hydraulic ==
  In1 : Inport
  Bus Selector : BusSelector  OutputSignals=signal1,signal2,signal3,signal4.H1_log,signal4.H2_log,signal4.H3_log
  Log Hydraulic System 1 Sensors : Subsystem  TreatAsAtomicUnit=on
  Log Hydraulic System 2 Sensors : Subsystem  TreatAsAtomicUnit=on
  Log Hydraulic System 3 Sensors : Subsystem  TreatAsAtomicUnit=on
  wires:
  [H1_log] -> Log Hydraulic System 1 Sensors/Enable
  In1/1 -> Bus Selector/1
  [H2_log] -> Log Hydraulic System 2 Sensors/Enable
  [H3_log] -> Log Hydraulic System 3 Sensors/Enable
  Bus Selector/1 -> Log Hydraulic System 1 Sensors/1(In1)  "<signal1>"
  Bus Selector/2 -> Log Hydraulic System 2 Sensors/1(In1)  "<signal2>"
  Bus Selector/3 -> Log Hydraulic System 3 Sensors/1(In1)  "<signal3>"
  Bus Selector/4 -> [H1_log]  "<H1_log>"
  Bus Selector/5 -> [H2_log]  "<H2_log>"
  Bus Selector/6 -> [H3_log]  "<H3_log>"

== system asbhl20/HL-20 Vehicle Systems Model/Avionics/Left Avionics Bay/CPU C/Event Logging/Event Logging Left ==
  In1 : Inport
  Bus Selector : BusSelector  OutputSignals=signal1,signal2,signal3,signal4,signal5.LU1_log,signal5.LU2_log,signal5.LL1_log,signal5.LL2_log
  Log LL1 Actuator Position Sensors : Subsystem  TreatAsAtomicUnit=on
  Log LL2 Actuator Position Sensors : Subsystem  TreatAsAtomicUnit=on
  Log LU1 Actuator Position Sensors : Subsystem  TreatAsAtomicUnit=on
  Log LU2 Actuator Position Sensors : Subsystem  TreatAsAtomicUnit=on
  wires:
  [LU1_log] -> Log LU1 Actuator Position Sensors/Enable
  In1/1 -> Bus Selector/1
  [LU2_log] -> Log LU2 Actuator Position Sensors/Enable
  [LL1_log] -> Log LL1 Actuator Position Sensors/Enable
  [LL2_log] -> Log LL2 Actuator Position Sensors/Enable
  Bus Selector/1 -> Log LU1 Actuator Position Sensors/1(In1)  "<signal1>"
  Bus Selector/2 -> Log LU2 Actuator Position Sensors/1(In1)  "<signal2>"
  Bus Selector/3 -> Log LL1 Actuator Position Sensors/1(In1)  "<signal3>"
  Bus Selector/4 -> Log LL2 Actuator Position Sensors/1(In1)  "<signal4>"
  Bus Selector/5 -> [LU1_log]  "<LU1_log>"
  Bus Selector/6 -> [LU2_log]  "<LU2_log>"
  Bus Selector/7 -> [LL1_log]  "<LL1_log>"
  Bus Selector/8 -> [LL2_log]  "<LL2_log>"

== system asbhl20/HL-20 Vehicle Systems Model/Avionics/Left Avionics Bay/CPU C/Event Logging/Event Logging Lower Hydraulic ==
  In1 : Inport
  Bus Selector : BusSelector  OutputSignals=signal1,signal2,signal3,signal4.H7_log,signal4.H8_log,signal4.H9_log
  Log Hydraulic System 1 Sensors : Subsystem  TreatAsAtomicUnit=on
  Log Hydraulic System 2 Sensors : Subsystem  TreatAsAtomicUnit=on
  Log Hydraulic System 3 Sensors : Subsystem  TreatAsAtomicUnit=on
  wires:
  [H7_log] -> Log Hydraulic System 1 Sensors/Enable
  In1/1 -> Bus Selector/1
  [H8_log] -> Log Hydraulic System 2 Sensors/Enable
  [H9_log] -> Log Hydraulic System 3 Sensors/Enable
  Bus Selector/1 -> Log Hydraulic System 1 Sensors/1(In1)  "<signal1>"
  Bus Selector/2 -> Log Hydraulic System 2 Sensors/1(In1)  "<signal2>"
  Bus Selector/3 -> Log Hydraulic System 3 Sensors/1(In1)  "<signal3>"
  Bus Selector/4 -> [H7_log]  "<H7_log>"
  Bus Selector/5 -> [H8_log]  "<H8_log>"
  Bus Selector/6 -> [H9_log]  "<H9_log>"

== system asbhl20/HL-20 Vehicle Systems Model/Avionics/Left Avionics Bay/CPU C/Event Logging/Event Logging Right ==
  In1 : Inport
  Bus Selector : BusSelector  OutputSignals=signal1,signal2,signal3,signal4,signal5.RU1_log,signal5.RU2_log,signal5.RL1_log,signal5.RL2_log
  Log RL1 Actuator Position Sensors : Subsystem  TreatAsAtomicUnit=on
  Log RL2 Actuator Position Sensors : Subsystem  TreatAsAtomicUnit=on
  Log RU1 Actuator Position Sensors : Subsystem  TreatAsAtomicUnit=on
  Log RU2 Actuator Position Sensors : Subsystem  TreatAsAtomicUnit=on
  wires:
  Bus Selector/4 -> Log RL2 Actuator Position Sensors/1(In1)  "<signal4>"
  Bus Selector/3 -> Log RL1 Actuator Position Sensors/1(In1)  "<signal3>"
  Bus Selector/2 -> Log RU2 Actuator Position Sensors/1(In1)  "<signal2>"
  Bus Selector/1 -> Log RU1 Actuator Position Sensors/1(In1)  "<signal1>"
  [RL2_log] -> Log RL2 Actuator Position Sensors/Enable
  [RL1_log] -> Log RL1 Actuator Position Sensors/Enable
  [RU2_log] -> Log RU2 Actuator Position Sensors/Enable
  In1/1 -> Bus Selector/1
  [RU1_log] -> Log RU1 Actuator Position Sensors/Enable
  Bus Selector/5 -> [RU1_log]  "<RU1_log>"
  Bus Selector/6 -> [RU2_log]  "<RU2_log>"
  Bus Selector/7 -> [RL1_log]  "<RL1_log>"
  Bus Selector/8 -> [RL2_log]  "<RL2_log>"

== system asbhl20/HL-20 Vehicle Systems Model/Avionics/Left Avionics Bay/CPU C/Event Logging/Event Logging Upper Hydraulic ==
  In1 : Inport
  Bus Selector : BusSelector  OutputSignals=signal1,signal2,signal3,signal4.H4_log,signal4.H5_log,signal4.H6_log
  Log Hydraulic System 1 Sensors : Subsystem  TreatAsAtomicUnit=on
  Log Hydraulic System 2 Sensors : Subsystem  TreatAsAtomicUnit=on
  Log Hydraulic System 3 Sensors : Subsystem  TreatAsAtomicUnit=on
  wires:
  Bus Selector/3 -> Log Hydraulic System 3 Sensors/1(In1)  "<signal3>"
  Bus Selector/2 -> Log Hydraulic System 2 Sensors/1(In1)  "<signal2>"
  Bus Selector/1 -> Log Hydraulic System 1 Sensors/1(In1)  "<signal1>"
  [H6_log] -> Log Hydraulic System 3 Sensors/Enable
  [H5_log] -> Log Hydraulic System 2 Sensors/Enable
  In1/1 -> Bus Selector/1
  [H4_log] -> Log Hydraulic System 1 Sensors/Enable
  Bus Selector/4 -> [H4_log]  "<H4_log>"
  Bus Selector/5 -> [H5_log]  "<H5_log>"
  Bus Selector/6 -> [H6_log]  "<H6_log>"
